simulink model "RBDmodel"  (R2023a)
settings: Solver=ode15s  StartTime=0.0  StopTime=4  FixedStep=0.0001  RelTol=1e-3  AbsTol=1e-3  EnableMultiTasking=on
model workspace (MAT data in the model file):
  C_Gimbal = 0.5
  C_IAP = 0.01
  IAP_Pa = 0
  K_Gimbal = 0
  K_IAP = 200
  LeftAbdominalMuscleForce = 0
  LeftBackMuscleForce = 0
  LeftTransverse1MuscleForce = 0
  LeftTransverse2MuscleForce = 0
  Moment_AR = 0
  Moment_FE = 7.5
  Moment_LB = 0
  RightAbdominalMuscleForce = 0
  RightBackMuscleForce = 0
  RightTransverse1MuscleForce = 0
  RightTransverse2MuscleForce = 0
  a = 1
  b = 1
  muscle_color = [0 0 1]
  muscle_radius = 1
undefined symbols (not defined in the file): X, Y, Z
libraries: nesl_utility x346, sm_lib x329, simulink_extras x33, checkpacklib x3, simulink x1
(part 8 of 12)

== system RBDmodel/main_model/L5 ==
  AR torque feedback L5 : Subsystem
  FE torque feedback L5 : Subsystem
  File Solid : sm_lib/Body Elements/File Solid  ExtGeomFileName=C:\Users\siril\OneDrive\Desktop\TIM-Control\Matlab\Simscape models\CAD - with COM\SymmetricModel\draft7\L5.step  UnitType=FromFile  ExtGeomFileUnits=m  StepReaderType=HEX  ExportConvexHullGeometry=off  InertiaType=CalculateFromGeometry  Mass=1  MassUnits=kg  CenterOfMass=[0 0 0]  CenterOfMassUnits=m  MomentsOfInertia=[1 1 1]  MomentsOfInertiaUnits=kg*m^2  ProductsOfInertia=[0 0 0]  ProductsOfInertiaUnits=kg*m^2  BasedOnType=Density  Density=0.182  DensityUnits=g/cm^3  DoExposeReferenceFrame=on  SerializedFrames=<Frames><Frame><Id>Frame1</Id><Value><Name>To Sacrum</Name><Origin><Source>GeometricFeature</Source><FeatureName>planar surface 1973</FeatureName></Origin><PrimaryAxis><DefinedDirection>+Z</DefinedDirection><Source>GeometricFeature</Source><SourceDirection>+Z</SourceDirection><FeatureName>planar surface 1973</FeatureName></PrimaryAxis><SecondaryAxis><DefinedDirection>+X</DefinedDirection><Source>ReferenceFrame</Source><SourceDirection>+X</SourceDirection><FeatureName></FeatureName></SecondaryAxis></Value></Frame><Frame><Id>Frame2</Id><Value><Name>To L4</Name><Origin><Source>GeometricFeature</Source><FeatureName>planar surface 1977</FeatureName></Origin><PrimaryAxis><DefinedDirection>+Z</DefinedDirection><Source>GeometricFeature</Source><SourceDirection>+Z</SourceDirection><FeatureName>planar surface 1977</FeatureName></PrimaryAxis><SecondaryAxis><DefinedDirection>+X</DefinedDirection><Source>ReferenceFrame</Source><SourceDirection>+X</SourceDirection><FeatureName></FeatureName></SecondaryAxis></Value></Frame><Frame><Id>Frame3</Id><Value><Name>L5 COM</Name><Origin><Source>CenterOfMassFrame</Source><FeatureName></FeatureName></Origin><PrimaryAxis><DefinedDirection>+Z</DefinedDirection><Source>ReferenceFrame</Source><SourceDirection>+Z</SourceDirection><FeatureName></FeatureName></PrimaryAxis><SecondaryAxis><DefinedDirection>+X</DefinedDirection><Source>ReferenceFrame</Source><SourceDirection>+X</SourceDirection><FeatureName></FeatureName></SecondaryAxis></Value></Frame><Frame><Id>Frame4</Id><Value><Name>L5 Abd Force</Name><Origin><Source>GeometricFeature</Source><FeatureName>point 2</FeatureName></Origin><PrimaryAxis><DefinedDirection>+Z</DefinedDirection><Source>GeometricFeature</Source><SourceDirection>+Z</SourceDirection><FeatureName>conical surface 1</FeatureName></PrimaryAxis><SecondaryAxis><DefinedDirection>+X</DefinedDirection><Source>ReferenceFrame</Source><SourceDirection>+X</SourceDirection><FeatureName></FeatureName></SecondaryAxis></Value></Frame><Frame><Id>Frame5</Id><Value><Name>To L4 ISL</Name><Origin><Source>GeometricFeature</Source><FeatureName>point 104</FeatureName></Origin><PrimaryAxis><DefinedDirection>+Z</DefinedDirection><Source>ReferenceFrame</Source><SourceDirection>+Z</SourceDirection><FeatureName></FeatureName></PrimaryAxis><SecondaryAxis><DefinedDirection>+X</DefinedDirection><Source>ReferenceFrame</Source><SourceDirection>+X</SourceDirection><FeatureName></FeatureName></SecondaryAxis></Value></Frame><Frame><Id>Frame6</Id><Value><Name>To S1 ISL</Name><Origin><Source>GeometricFeature</Source><FeatureName>point 11405</FeatureName></Origin><PrimaryAxis><DefinedDirection>+Z</DefinedDirection><Source>ReferenceFrame</Source><SourceDirection>+Z</SourceDirection><FeatureName></FeatureName></PrimaryAxis><SecondaryAxis><DefinedDirection>+X</DefinedDirection><Source>ReferenceFrame</Source><SourceDirection>+X</SourceDirection><FeatureName></FeatureName></SecondaryAxis></Value></Frame><Frame><Id>Frame7</Id><Value><Name>To S1 SSL</Name><Origin><Source>GeometricFeature</Source><FeatureName>point 8728</FeatureName></Origin><PrimaryAxis><DefinedDirection>+Z</DefinedDirection><Source>ReferenceFrame</Source><SourceDirection>+Z</SourceDirection><FeatureName></FeatureName></PrimaryAxis><SecondaryAxis><DefinedDirection>+X</DefinedDirection><Source>ReferenceFrame</Source><SourceDirection>+X</SourceDirection><FeatureName></FeatureName></SecondaryAxis></Value></Frame><Frame><Id>Frame8</Id><Value><Name>To L4 SSL</Name><Origin><Source>GeometricFeature</Source><FeatureName>point 5958</FeatureName></Origin><PrimaryAxis><DefinedDirection>+Z</DefinedDirection><Source>ReferenceFrame</Source><SourceDirection>+Z</SourceDirection><FeatureName></FeatureName></PrimaryAxis><SecondaryAxis><DefinedDirection>+X</DefinedDirection><Source>ReferenceFrame</Source><SourceDirection>+X</SourceDirection><FeatureName></FeatureName></SecondaryAxis></Value></Frame><Frame><Id>Frame9</Id><Value><Name>To Left S1 ITL</Name><Origin><Source>GeometricFeature</Source><FeatureName>point 9071</FeatureName></Origin><PrimaryAxis><DefinedDirection>+Z</DefinedDirection><Source>ReferenceFrame</Source><SourceDirection>+Z</SourceDirection><FeatureName></FeatureName></PrimaryAxis><SecondaryAxis><DefinedDirection>+X</DefinedDirection><Source>ReferenceFrame</Source><SourceDirection>+X</SourceDirection><FeatureName></FeatureName></SecondaryAxis></Value></Frame><Frame><Id>Frame10</Id><Value><Name>To Right S1 ITL</Name><Origin><Source>GeometricFeature</Source><FeatureName>point 3312</FeatureName></Origin><PrimaryAxis><DefinedDirection>+Z</DefinedDirection><Source>ReferenceFrame</Source><SourceDirection>+Z</SourceDirection><FeatureName></FeatureName></PrimaryAxis><SecondaryAxis><DefinedDirection>+X</DefinedDirection><Source>ReferenceFrame</Source><SourceDirection>+X</SourceDirection><FeatureName></FeatureName></SecondaryAxis></Value></Frame><Frame><Id>Frame11</Id><Value><Name>To Left L4 ITL</Name><Origin><Source>GeometricFeature</Source><FeatureName>point 10699</FeatureName></Origin><PrimaryAxis><DefinedDirection>+Z</DefinedDirection><Source>ReferenceFrame</Source><SourceDirection>+Z</SourceDirection><FeatureName></FeatureName></PrimaryAxis><SecondaryAxis><DefinedDirection>+X</DefinedDirection><Source>ReferenceFrame</Source><SourceDirection>+X</SourceDirection><FeatureName></FeatureName></SecondaryAxis></Value></Frame><Frame><Id>Frame12</Id><Value><Name>To Right L4 ITL</Name><Origin><Source>GeometricFeature</Source><FeatureName>point 5014</FeatureName></Origin><PrimaryAxis><DefinedDirection>+Z</DefinedDirection><Source>ReferenceFrame</Source><SourceDirection>+Z</SourceDirection><FeatureName></FeatureName></PrimaryAxis><SecondaryAxis><DefinedDirection>+X</DefinedDirection><Source>ReferenceFrame</Source><SourceDirection>+X</SourceDirection><FeatureName></FeatureName></SecondaryAxis></Value></Frame></Frames>  GraphicType=FromGeometry  MarkerShape=Sphere  MarkerSize=10  GraphicVisPropType=SimpleVisualProperties  GraphicDiffuseColor=[0.8901961 0.85490197 0.7882353]  GraphicSpecularColor=[0.5 0.5 0.5 1.0]  GraphicAmbientColor=[0.15 0.15 0.15 1.0]  GraphicEmissiveColor=[0.0 0.0 0.0 1.0]  GraphicShininess=75  GraphicOpacity=1.0
  Gimbal Joint : sm_lib/Joints/Gimbal Joint  JointMode=Normal  SenseConstraintForce=on  SenseConstraintForceX=off  SenseConstraintForceY=off  SenseConstraintForceZ=off  SenseConstraintTorque=off  SenseConstraintTorqueX=off  SenseConstraintTorqueY=off  SenseConstraintTorqueZ=off  SenseTotalForce=on  SenseTotalForceX=off  SenseTotalForceY=off  SenseTotalForceZ=off  SenseTotalTorque=off  SenseTotalTorqueX=off  SenseTotalTorqueY=off  SenseTotalTorqueZ=off  CompositeWrenchDir=FollowerOnBase  CompositeWrenchFrame=BaseFrame  RxEquilibriumPosition=0  RxEquilibriumPositionUnits=deg  RxSpringStiffness=K_Gimbal  RxSpringStiffnessUnits=N*m/deg  RxDampingCoefficient=C_Gimbal  RxDampingCoefficientUnits=N*m/(deg/s)  RxTorqueActuationMode=InputTorque  RxMotionActuationMode=ComputedMotion  RxSensePosition=on  RxSenseVelocity=off  RxSenseAcceleration=off  RxSenseTorqueForce=on  RxSenseLowerLimitTorqueForce=off  RxSenseUpperLimitTorqueForce=off  RxLowerLimitSpecify=on  RxLowerLimitBound=-30  RxLowerLimitBoundUnits=deg  RxLowerLimitStiffness=10000  RxLowerLimitStiffnessUnits=N*m/deg  RxLowerLimitDamping=100  RxLowerLimitDampingUnits=N*m/(deg/s)  RxLowerLimitTransitionRegionWidth=0.1  RxLowerLimitTransitionRegionWidthUnits=deg  RxUpperLimitSpecify=on  RxUpperLimitBound=30  RxUpperLimitBoundUnits=deg  RxUpperLimitStiffness=10000  RxUpperLimitStiffnessUnits=N*m/deg  RxUpperLimitDamping=100  RxUpperLimitDampingUnits=N*m/(deg/s)  RxUpperLimitTransitionRegionWidth=0.1  RxUpperLimitTransitionRegionWidthUnits=deg  RxPositionTargetSpecify=off  RxPositionTargetPriority=High  RxPositionTargetValue=0  RxPositionTargetValueUnits=deg  RxVelocityTargetSpecify=off  RxVelocityTargetPriority=High  RxVelocityTargetValue=0  RxVelocityTargetValueUnits=deg/s  RyEquilibriumPosition=0  RyEquilibriumPositionUnits=deg  RySpringStiffness=K_Gimbal  RySpringStiffnessUnits=N*m/deg  RyDampingCoefficient=C_Gimbal  RyDampingCoefficientUnits=N*m/(deg/s)  RyTorqueActuationMode=InputTorque  RyMotionActuationMode=ComputedMotion  RySensePosition=on  RySenseVelocity=off  RySenseAcceleration=off  RySenseTorqueForce=on  RySenseLowerLimitTorqueForce=off  RySenseUpperLimitTorqueForce=off  RyLowerLimitSpecify=on  RyLowerLimitBound=-30  RyLowerLimitBoundUnits=deg  RyLowerLimitStiffness=10000  RyLowerLimitStiffnessUnits=N*m/deg  RyLowerLimitDamping=100  RyLowerLimitDampingUnits=N*m/(deg/s)  RyLowerLimitTransitionRegionWidth=0.1  RyLowerLimitTransitionRegionWidthUnits=deg  RyUpperLimitSpecify=on  RyUpperLimitBound=30  RyUpperLimitBoundUnits=deg  RyUpperLimitStiffness=10000  RyUpperLimitStiffnessUnits=N*m/deg  RyUpperLimitDamping=100  RyUpperLimitDampingUnits=N*m/(deg/s)  RyUpperLimitTransitionRegionWidth=0.1  RyUpperLimitTransitionRegionWidthUnits=deg  RyPositionTargetSpecify=off  RyPositionTargetPriority=High  RyPositionTargetValue=0  RyPositionTargetValueUnits=deg  RyVelocityTargetSpecify=off  RyVelocityTargetPriority=High  RyVelocityTargetValue=0  RyVelocityTargetValueUnits=deg/s  RzEquilibriumPosition=0  RzEquilibriumPositionUnits=deg  RzSpringStiffness=K_Gimbal  RzSpringStiffnessUnits=N*m/deg  RzDampingCoefficient=C_Gimbal  RzDampingCoefficientUnits=N*m/(deg/s)  RzTorqueActuationMode=InputTorque  RzMotionActuationMode=ComputedMotion  RzSensePosition=on  RzSenseVelocity=off  RzSenseAcceleration=off  RzSenseTorqueForce=on  RzSenseLowerLimitTorqueForce=off  RzSenseUpperLimitTorqueForce=off  RzLowerLimitSpecify=on  RzLowerLimitBound=-30  RzLowerLimitBoundUnits=deg  RzLowerLimitStiffness=10000  RzLowerLimitStiffnessUnits=N*m/deg  RzLowerLimitDamping=100  RzLowerLimitDampingUnits=N*m/(deg/s)  RzLowerLimitTransitionRegionWidth=0.1  RzLowerLimitTransitionRegionWidthUnits=deg  RzUpperLimitSpecify=on  RzUpperLimitBound=30  RzUpperLimitBoundUnits=deg  RzUpperLimitStiffness=10000  RzUpperLimitStiffnessUnits=N*m/deg  RzUpperLimitDamping=100  RzUpperLimitDampingUnits=N*m/(deg/s)  RzUpperLimitTransitionRegionWidth=0.1  RzUpperLimitTransitionRegionWidthUnits=deg  RzPositionTargetSpecify=off  RzPositionTargetPriority=High  RzPositionTargetValue=0  RzPositionTargetValueUnits=deg  RzVelocityTargetSpecify=off  RzVelocityTargetPriority=High  RzVelocityTargetValue=0  RzVelocityTargetValueUnits=deg/s
  LB torque feedback L5 : Subsystem
  to sacrum : PMIOPort  Side=Left
  to L4 : PMIOPort  Port=2  Side=Right
  FE torque : PMIOPort  Port=3  Side=Right
  FE rot : PMIOPort  Port=4  Side=Right
  LB rot : PMIOPort  Port=5  Side=Right
  LB torque : PMIOPort  Port=6  Side=Right
  AR rot : PMIOPort  Port=7  Side=Right
  AR torque : PMIOPort  Port=8  Side=Right
  L5 COM : PMIOPort  Port=9  Side=Right
  L5 Abd Force : PMIOPort  Port=10  Side=Right
  To L4 ISL : PMIOPort  Port=11  Side=Right
  To S1 ISL : PMIOPort  Port=12  Side=Right
  To L4 SSL : PMIOPort  Port=13  Side=Right
  To S1 SSL : PMIOPort  Port=14  Side=Right
  To Left S1 ITL : PMIOPort  Port=15  Side=Right
  To Right S1 ITL : PMIOPort  Port=16  Side=Right
  To Left L4 ITL : PMIOPort  Port=17  Side=Right
  To Right L4 ITL : PMIOPort  Port=18  Side=Right
  connections:
  File Solid/LConn2 -- to L4/RConn1
  to sacrum/RConn1 -- Gimbal Joint/LConn1
  Gimbal Joint/RConn1 -- File Solid/LConn1
  Gimbal Joint/LConn2 -- FE torque feedback L5/RConn1
  Gimbal Joint/LConn3 -- LB torque feedback L5/RConn1
  Gimbal Joint/LConn4 -- AR torque feedback L5/RConn1
  Gimbal Joint/RConn2 -- FE torque feedback L5/LConn1 -- FE rot/RConn1
  Gimbal Joint/RConn4 -- LB torque feedback L5/LConn1 -- LB rot/RConn1
  Gimbal Joint/RConn6 -- AR rot/RConn1 -- AR torque feedback L5/LConn1
  FE torque/RConn1 -- Gimbal Joint/RConn3
  LB torque/RConn1 -- Gimbal Joint/RConn5
  AR torque/RConn1 -- Gimbal Joint/RConn7
  L5 COM/RConn1 -- File Solid/RConn2
  L5 Abd Force/RConn1 -- File Solid/LConn3
  To L4 ISL/RConn1 -- File Solid/RConn3
  To S1 ISL/RConn1 -- File Solid/LConn4
  To S1 SSL/RConn1 -- File Solid/RConn4
  To L4 SSL/RConn1 -- File Solid/LConn5
  To Left S1 ITL/RConn1 -- File Solid/RConn5
  To Right S1 ITL/RConn1 -- File Solid/LConn6
  To Left L4 ITL/RConn1 -- File Solid/RConn6
  To Right L4 ITL/RConn1 -- File Solid/LConn7

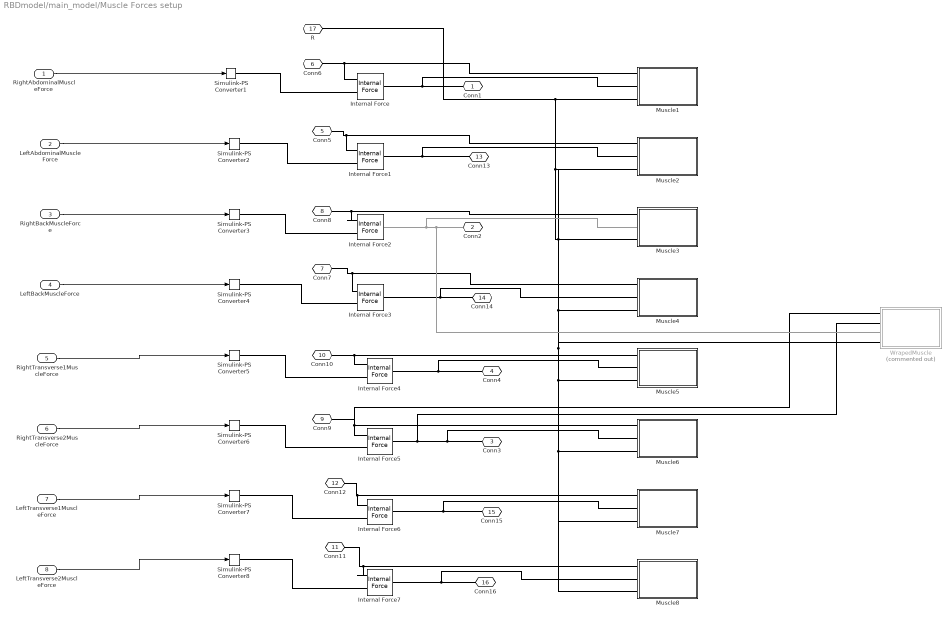
== system RBDmodel/main_model/Muscle Forces setup ==
  RightAbdominalMuscleForce : Inport
  LeftAbdominalMuscleForce : Inport  Port=2
  RightBackMuscleForce : Inport  Port=3
  LeftBackMuscleForce : Inport  Port=4
  RightTransverse1MuscleForce : Inport  Port=5
  RightTransverse2MuscleForce : Inport  Port=6
  LeftTransverse1MuscleForce : Inport  Port=7
  LeftTransverse2MuscleForce : Inport  Port=8
  Internal Force{,1..7} (8 alike) : sm_lib/Forces and Torques/Internal Force
  Muscle1 : Subsystem
  Muscle2 : Subsystem
  Muscle3 : Subsystem
  Muscle4 : Subsystem
  Muscle5 : Subsystem
  Muscle6 : Subsystem
  Muscle7 : Subsystem
  Muscle8 : Subsystem
  Simulink-PS Converter{1..8} (8 alike) : nesl_utility/Simulink-PS Converter  PhysicalDomain=network_engine_domain  SubClassName=ps_input  LeftPortType=input  RightPortType=output  PseudoPeriodic=off  Frequencies=[]  NoiseDistribution=none  NoiseParameters=[]  Unit=1  AffineConversion=off  FilteringAndDerivatives=provide  SimscapeFilterOrder=1  InputFilterTimeConstant=0.001  UdotUserProvided=0
  WrapedMuscle : Subsystem  Commented=on
  Conn1 : PMIOPort  Side=Right
  Conn2 : PMIOPort  Port=2  Side=Right
  Conn3 : PMIOPort  Port=3  Side=Right
  Conn4 : PMIOPort  Port=4  Side=Right
  Conn5 : PMIOPort  Port=5  Side=Left
  Conn6 : PMIOPort  Port=6  Side=Left
  Conn7 : PMIOPort  Port=7  Side=Left
  Conn8 : PMIOPort  Port=8  Side=Left
  Conn9 : PMIOPort  Port=9  Side=Left
  Conn10 : PMIOPort  Port=10  Side=Left
  Conn11 : PMIOPort  Port=11  Side=Left
  Conn12 : PMIOPort  Port=12  Side=Left
  Conn13 : PMIOPort  Port=13  Side=Right
  Conn14 : PMIOPort  Port=14  Side=Right
  Conn15 : PMIOPort  Port=15  Side=Right
  Conn16 : PMIOPort  Port=16  Side=Right
  R : PMIOPort  Port=17  Side=Left
  wires:
  LeftTransverse2MuscleForce/1 -> Simulink-PS Converter8/1
  RightBackMuscleForce/1 -> Simulink-PS Converter3/1
  RightTransverse1MuscleForce/1 -> Simulink-PS Converter5/1
  LeftTransverse1MuscleForce/1 -> Simulink-PS Converter7/1
  RightTransverse2MuscleForce/1 -> Simulink-PS Converter6/1
  LeftAbdominalMuscleForce/1 -> Simulink-PS Converter2/1
  RightAbdominalMuscleForce/1 -> Simulink-PS Converter1/1
  LeftBackMuscleForce/1 -> Simulink-PS Converter4/1
  connections:
  Muscle4/RConn1 -- Conn7/RConn1 -- Internal Force3/LConn1
  Conn9/RConn1 -- WrapedMuscle/RConn1 -- Muscle6/RConn1 -- Internal Force5/LConn1
  Muscle8/RConn3 -- Muscle7/RConn3 -- Muscle6/RConn3 -- Muscle5/RConn3 -- WrapedMuscle/RConn4 -- Muscle4/RConn3 -- Muscle3/RConn3 -- Muscle2/RConn3 -- R/RConn1 -- Muscle1/RConn3
  Muscle4/RConn2 -- Conn14/RConn1 -- Internal Force3/RConn1
  Muscle5/RConn1 -- Conn10/RConn1 -- Internal Force4/LConn1
  Muscle6/RConn2 -- Conn3/RConn1 -- WrapedMuscle/RConn2 -- Internal Force5/RConn1
  Muscle7/RConn1 -- Conn12/RConn1 -- Internal Force6/LConn1
  Internal Force7/LConn1 -- Conn11/RConn1 -- Muscle8/RConn1
  Simulink-PS Converter8/RConn1 -- Internal Force7/LConn2
  Muscle2/RConn1 -- Conn5/RConn1 -- Internal Force1/LConn1
  Simulink-PS Converter2/RConn1 -- Internal Force1/LConn2
  Muscle7/RConn2 -- Conn15/RConn1 -- Internal Force6/RConn1
  Muscle2/RConn2 -- Conn13/RConn1 -- Internal Force1/RConn1
  Simulink-PS Converter1/RConn1 -- Internal Force/LConn2
  WrapedMuscle/RConn3 -- Conn2/RConn1 -- Muscle3/RConn2 -- Internal Force2/RConn1
  Muscle1/RConn1 -- Conn6/RConn1 -- Internal Force/LConn1
  Simulink-PS Converter3/RConn1 -- Internal Force2/LConn2
  Simulink-PS Converter7/RConn1 -- Internal Force6/LConn2
  Internal Force2/LConn1 -- Conn8/RConn1 -- Muscle3/RConn1
  Muscle1/RConn2 -- Conn1/RConn1 -- Internal Force/RConn1
  Simulink-PS Converter5/RConn1 -- Internal Force4/LConn2
  Muscle8/RConn2 -- Conn16/RConn1 -- Internal Force7/RConn1
  Muscle5/RConn2 -- Conn4/RConn1 -- Internal Force4/RConn1
  Simulink-PS Converter4/RConn1 -- Internal Force3/LConn2
  Simulink-PS Converter6/RConn1 -- Internal Force5/LConn2

== system RBDmodel/main_model/Plumbline setup ==
  Gain : Gain  Gain=100
  Gain1 : Gain  Gain=100
  Gain2 : Gain  Gain=100
  PS-Simulink Converter2 : nesl_utility/PS-Simulink Converter  PhysicalDomain=network_engine_domain  SubClassName=ps_output  LeftPortType=input  RightPortType=output  PseudoPeriodic=off  Frequencies=[]  VectorFormat=inherit  Unit=inherit  AffineConversion=off
  PS-Simulink Converter3 : nesl_utility/PS-Simulink Converter  PhysicalDomain=network_engine_domain  SubClassName=ps_output  LeftPortType=input  RightPortType=output  PseudoPeriodic=off  Frequencies=[]  VectorFormat=inherit  Unit=inherit  AffineConversion=off
  PS-Simulink Converter4 : nesl_utility/PS-Simulink Converter  PhysicalDomain=network_engine_domain  SubClassName=ps_output  LeftPortType=input  RightPortType=output  PseudoPeriodic=off  Frequencies=[]  VectorFormat=inherit  Unit=inherit  AffineConversion=off
  T1-S1 Bushing Joint : sm_lib/Joints/Bushing Joint  JointMode=Normal  SenseConstraintForce=off  SenseConstraintForceX=off  SenseConstraintForceY=off  SenseConstraintForceZ=off  SenseConstraintTorque=off  SenseConstraintTorqueX=off  SenseConstraintTorqueY=off  SenseConstraintTorqueZ=off  SenseTotalForce=off  SenseTotalForceX=off  SenseTotalForceY=off  SenseTotalForceZ=off  SenseTotalTorque=off  SenseTotalTorqueX=off  SenseTotalTorqueY=off  SenseTotalTorqueZ=off  CompositeWrenchDir=FollowerOnBase  CompositeWrenchFrame=BaseFrame  PxEquilibriumPosition=0  PxEquilibriumPositionUnits=m  PxSpringStiffness=0  PxSpringStiffnessUnits=N/m  PxDampingCoefficient=0  PxDampingCoefficientUnits=N/(m/s)  PxTorqueActuationMode=NoTorque  PxMotionActuationMode=ComputedMotion  PxSensePosition=on  PxSenseVelocity=off  PxSenseAcceleration=off  PxSenseTorqueForce=off  PxSenseLowerLimitTorqueForce=off  PxSenseUpperLimitTorqueForce=off  PxLowerLimitSpecify=off  PxLowerLimitBound=-1  PxLowerLimitBoundUnits=m  PxLowerLimitStiffness=1e6  PxLowerLimitStiffnessUnits=N/m  PxLowerLimitDamping=1e3  PxLowerLimitDampingUnits=N/(m/s)  PxLowerLimitTransitionRegionWidth=1e-4  PxLowerLimitTransitionRegionWidthUnits=m  PxUpperLimitSpecify=off  PxUpperLimitBound=1  PxUpperLimitBoundUnits=m  PxUpperLimitStiffness=1e6  PxUpperLimitStiffnessUnits=N/m  PxUpperLimitDamping=1e3  PxUpperLimitDampingUnits=N/(m/s)  PxUpperLimitTransitionRegionWidth=1e-4  PxUpperLimitTransitionRegionWidthUnits=m  PxPositionTargetSpecify=off  PxPositionTargetPriority=High  PxPositionTargetValue=0  PxPositionTargetValueUnits=m  PxVelocityTargetSpecify=off  PxVelocityTargetPriority=High  PxVelocityTargetValue=0  PxVelocityTargetValueUnits=m/s  PyEquilibriumPosition=0  PyEquilibriumPositionUnits=m  PySpringStiffness=0  PySpringStiffnessUnits=N/m  PyDampingCoefficient=0  PyDampingCoefficientUnits=N/(m/s)  PyTorqueActuationMode=NoTorque  PyMotionActuationMode=ComputedMotion  PySensePosition=on  PySenseVelocity=off  PySenseAcceleration=off  PySenseTorqueForce=off  PySenseLowerLimitTorqueForce=off  PySenseUpperLimitTorqueForce=off  PyLowerLimitSpecify=off  PyLowerLimitBound=-1  PyLowerLimitBoundUnits=m  PyLowerLimitStiffness=1e6  PyLowerLimitStiffnessUnits=N/m  PyLowerLimitDamping=1e3  PyLowerLimitDampingUnits=N/(m/s)  PyLowerLimitTransitionRegionWidth=1e-4  PyLowerLimitTransitionRegionWidthUnits=m  PyUpperLimitSpecify=off  PyUpperLimitBound=1  PyUpperLimitBoundUnits=m  PyUpperLimitStiffness=1e6  PyUpperLimitStiffnessUnits=N/m  PyUpperLimitDamping=1e3  PyUpperLimitDampingUnits=N/(m/s)  PyUpperLimitTransitionRegionWidth=1e-4  PyUpperLimitTransitionRegionWidthUnits=m  PyPositionTargetSpecify=off  PyPositionTargetPriority=High  PyPositionTargetValue=0  PyPositionTargetValueUnits=m  PyVelocityTargetSpecify=off  PyVelocityTargetPriority=High  PyVelocityTargetValue=0  PyVelocityTargetValueUnits=m/s  PzEquilibriumPosition=0  PzEquilibriumPositionUnits=m  PzSpringStiffness=0  PzSpringStiffnessUnits=N/m  PzDampingCoefficient=0  PzDampingCoefficientUnits=N/(m/s)  PzTorqueActuationMode=NoTorque  PzMotionActuationMode=ComputedMotion  PzSensePosition=on  PzSenseVelocity=off  PzSenseAcceleration=off  PzSenseTorqueForce=off  PzSenseLowerLimitTorqueForce=off  PzSenseUpperLimitTorqueForce=off  PzLowerLimitSpecify=off  PzLowerLimitBound=-1  PzLowerLimitBoundUnits=m  PzLowerLimitStiffness=1e6  PzLowerLimitStiffnessUnits=N/m  PzLowerLimitDamping=1e3  PzLowerLimitDampingUnits=N/(m/s)  PzLowerLimitTransitionRegionWidth=1e-4  PzLowerLimitTransitionRegionWidthUnits=m  PzUpperLimitSpecify=off  PzUpperLimitBound=1  PzUpperLimitBoundUnits=m  PzUpperLimitStiffness=1e6  PzUpperLimitStiffnessUnits=N/m  PzUpperLimitDamping=1e3  PzUpperLimitDampingUnits=N/(m/s)  PzUpperLimitTransitionRegionWidth=1e-4  PzUpperLimitTransitionRegionWidthUnits=m  PzPositionTargetSpecify=off  PzPositionTargetPriority=High  PzPositionTargetValue=0  PzPositionTargetValueUnits=m  PzVelocityTargetSpecify=off  PzVelocityTargetPriority=High  PzVelocityTargetValue=0  PzVelocityTargetValueUnits=m/s  RxEquilibriumPosition=0  RxEquilibriumPositionUnits=deg  RxSpringStiffness=0  RxSpringStiffnessUnits=N*m/deg  RxDampingCoefficient=0  RxDampingCoefficientUnits=N*m/(deg/s)  RxTorqueActuationMode=NoTorque  RxMotionActuationMode=ComputedMotion  RxSensePosition=off  RxSenseVelocity=off  RxSenseAcceleration=off  RxSenseTorqueForce=off  RxSenseLowerLimitTorqueForce=off  RxSenseUpperLimitTorqueForce=off  RxLowerLimitSpecify=off  RxLowerLimitBound=-90  RxLowerLimitBoundUnits=deg  RxLowerLimitStiffness=1e4  RxLowerLimitStiffnessUnits=N*m/deg  RxLowerLimitDamping=10  RxLowerLimitDampingUnits=N*m/(deg/s)  RxLowerLimitTransitionRegionWidth=0.1  RxLowerLimitTransitionRegionWidthUnits=deg  RxUpperLimitSpecify=off  RxUpperLimitBound=90  RxUpperLimitBoundUnits=deg  RxUpperLimitStiffness=1e4  RxUpperLimitStiffnessUnits=N*m/deg  RxUpperLimitDamping=10  RxUpperLimitDampingUnits=N*m/(deg/s)  RxUpperLimitTransitionRegionWidth=0.1  RxUpperLimitTransitionRegionWidthUnits=deg  RxPositionTargetSpecify=off  RxPositionTargetPriority=High  RxPositionTargetValue=0  RxPositionTargetValueUnits=deg  RxVelocityTargetSpecify=off  RxVelocityTargetPriority=High  RxVelocityTargetValue=0  RxVelocityTargetValueUnits=deg/s  RyEquilibriumPosition=0  RyEquilibriumPositionUnits=deg  RySpringStiffness=0  RySpringStiffnessUnits=N*m/deg  RyDampingCoefficient=0  RyDampingCoefficientUnits=N*m/(deg/s)  RyTorqueActuationMode=NoTorque  RyMotionActuationMode=ComputedMotion  RySensePosition=off  RySenseVelocity=off  RySenseAcceleration=off  RySenseTorqueForce=off  RySenseLowerLimitTorqueForce=off  RySenseUpperLimitTorqueForce=off  RyLowerLimitSpecify=off  RyLowerLimitBound=-90  RyLowerLimitBoundUnits=deg  RyLowerLimitStiffness=1e4  RyLowerLimitStiffnessUnits=N*m/deg  RyLowerLimitDamping=10  RyLowerLimitDampingUnits=N*m/(deg/s)  RyLowerLimitTransitionRegionWidth=0.1  RyLowerLimitTransitionRegionWidthUnits=deg  RyUpperLimitSpecify=off  RyUpperLimitBound=90  RyUpperLimitBoundUnits=deg  RyUpperLimitStiffness=1e4  RyUpperLimitStiffnessUnits=N*m/deg  RyUpperLimitDamping=10  RyUpperLimitDampingUnits=N*m/(deg/s)  RyUpperLimitTransitionRegionWidth=0.1  RyUpperLimitTransitionRegionWidthUnits=deg  RyPositionTargetSpecify=off  RyPositionTargetPriority=High  RyPositionTargetValue=0  RyPositionTargetValueUnits=deg  RyVelocityTargetSpecify=off  RyVelocityTargetPriority=High  RyVelocityTargetValue=0  RyVelocityTargetValueUnits=deg/s  RzEquilibriumPosition=0  RzEquilibriumPositionUnits=deg  RzSpringStiffness=0  RzSpringStiffnessUnits=N*m/deg  RzDampingCoefficient=0  RzDampingCoefficientUnits=N*m/(deg/s)  RzTorqueActuationMode=NoTorque  RzMotionActuationMode=ComputedMotion  RzSensePosition=off  RzSenseVelocity=off  RzSenseAcceleration=off  RzSenseTorqueForce=off  RzSenseLowerLimitTorqueForce=off  RzSenseUpperLimitTorqueForce=off  RzLowerLimitSpecify=off  RzLowerLimitBound=-90  RzLowerLimitBoundUnits=deg  RzLowerLimitStiffness=1e4  RzLowerLimitStiffnessUnits=N*m/deg  RzLowerLimitDamping=10  RzLowerLimitDampingUnits=N*m/(deg/s)  RzLowerLimitTransitionRegionWidth=0.1  RzLowerLimitTransitionRegionWidthUnits=deg  RzUpperLimitSpecify=off  RzUpperLimitBound=90  RzUpperLimitBoundUnits=deg  RzUpperLimitStiffness=1e4  RzUpperLimitStiffnessUnits=N*m/deg  RzUpperLimitDamping=10  RzUpperLimitDampingUnits=N*m/(deg/s)  RzUpperLimitTransitionRegionWidth=0.1  RzUpperLimitTransitionRegionWidthUnits=deg  RzPositionTargetSpecify=off  RzPositionTargetPriority=High  RzPositionTargetValue=0  RzPositionTargetValueUnits=deg  RzVelocityTargetSpecify=off  RzVelocityTargetPriority=High  RzVelocityTargetValue=0  RzVelocityTargetValueUnits=deg/s
  Conn1 : PMIOPort  Side=Left
  Conn2 : PMIOPort  Port=2  Side=Right
  x : Outport
  y : Outport  Port=2
  z : Outport  Port=3
  wires:
  PS-Simulink Converter3/1 -> Gain1/1  "y"
  Gain1/1 -> y/1  "y"
  PS-Simulink Converter2/1 -> Gain/1  "x"
  PS-Simulink Converter4/1 -> Gain2/1  "z"
  Gain/1 -> x/1  "x"
  Gain2/1 -> z/1  "z"
  connections:
  PS-Simulink Converter3/LConn1 -- T1-S1 Bushing Joint/RConn3
  PS-Simulink Converter4/LConn1 -- T1-S1 Bushing Joint/RConn4
  PS-Simulink Converter2/LConn1 -- T1-S1 Bushing Joint/RConn2
  Conn1/RConn1 -- T1-S1 Bushing Joint/LConn1
  T1-S1 Bushing Joint/RConn1 -- Conn2/RConn1

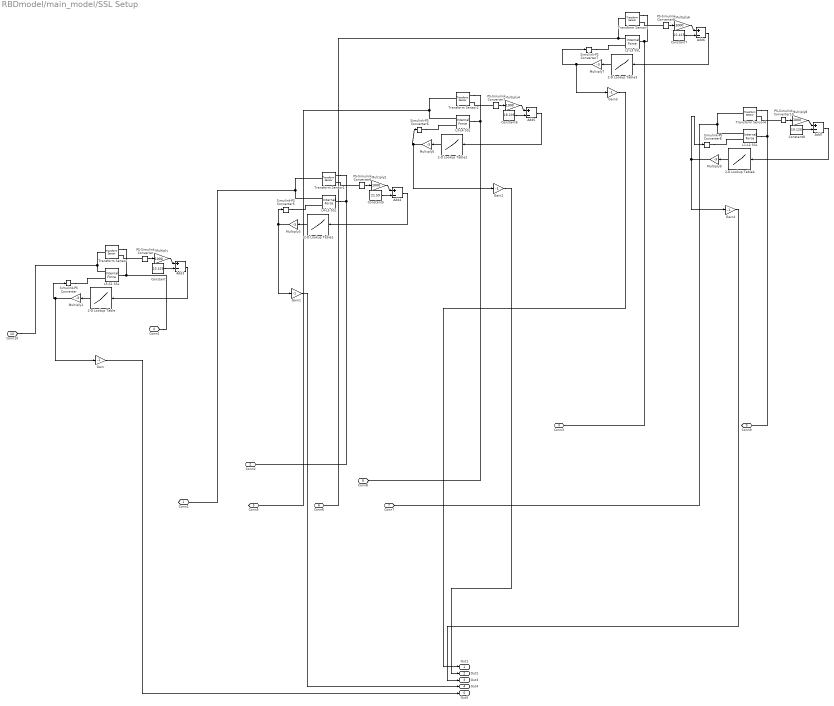
== system RBDmodel/main_model/SSL Setup ==
  2-D Lookup Table : Lookup_n-D  NumberOfTableDimensions=1  BreakpointsForDimension1=[0;0.272;4.08;5.984;7.888]  BreakpointsForDimension2=[1:3]  Table=[0;0;8.4;21;84]  InternalRulePriority=Speed  RndMeth=Simplest
  2-D Lookup Table1 : Lookup_n-D  NumberOfTableDimensions=1  BreakpointsForDimension1=[0;0.223;3.345;4.906;6.467]  BreakpointsForDimension2=[1:3]  Table=[0;0;8.4;21;84]  InternalRulePriority=Speed  RndMeth=Simplest
  2-D Lookup Table2 : Lookup_n-D  NumberOfTableDimensions=1  BreakpointsForDimension1=[0;0.194;2.91;4.268;5.626]  BreakpointsForDimension2=[1:3]  Table=[0;0;8.4;21;84]  InternalRulePriority=Speed  RndMeth=Simplest
  2-D Lookup Table3 : Lookup_n-D  NumberOfTableDimensions=1  BreakpointsForDimension1=[0;0.268;4.02;5.896;7.772]  BreakpointsForDimension2=[1:3]  Table=[0;0;8.4;21;84]  InternalRulePriority=Speed  RndMeth=Simplest
  2-D Lookup Table4 : Lookup_n-D  NumberOfTableDimensions=1  BreakpointsForDimension1=[0;0.223;3.345;4.906;6.467]  BreakpointsForDimension2=[1:3]  Table=[0;0;8.4;21;84]  InternalRulePriority=Speed  RndMeth=Simplest
  Add{3..7} (5 alike) : Sum  Inputs=+-
  Constant : Constant  Value=23.426
  Constant5 : Constant  Value=21.59
  Constant6 : Constant  Value=18.205
  Constant7 : Constant  Value=21.415
  Constant8 : Constant  Value=19.125
  Gain{,1..4} (5 alike) : Gain  Gain=-1
  L1-L2 SSL : sm_lib/Forces and Torques/Internal Force
  L2-L3 SSL : sm_lib/Forces and Torques/Internal Force
  L3-L4 SSL : sm_lib/Forces and Torques/Internal Force
  L4-L5 SSL : sm_lib/Forces and Torques/Internal Force
  L5-S1 SSL : sm_lib/Forces and Torques/Internal Force
  Multiply{,2,4,6,8} (5 alike) : Gain  Gain=1000
  Multiply{1,3,5,7,9} (5 alike) : Gain  Gain=-3
  PS-Simulink Converter{,6..8,10} (5 alike) : nesl_utility/PS-Simulink Converter  PhysicalDomain=network_engine_domain  SubClassName=ps_output  LeftPortType=input  RightPortType=output  PseudoPeriodic=off  Frequencies=[]  VectorFormat=inherit  Unit=inherit  AffineConversion=off
  Simulink-PS Converter{,5..8} (5 alike) : nesl_utility/Simulink-PS Converter  PhysicalDomain=network_engine_domain  SubClassName=ps_input  LeftPortType=input  RightPortType=output  PseudoPeriodic=off  Frequencies=[]  NoiseDistribution=none  NoiseParameters=[]  Unit=1  AffineConversion=off  FilteringAndDerivatives=provide  SimscapeFilterOrder=1  InputFilterTimeConstant=0.001  UdotUserProvided=0
  Transform Sensor{,1..4} (5 alike) : sm_lib/Frames and Transforms/Transform Sensor  MeasurementFrame=World  RotationSequence=XYX  SenseAngle=off  SenseAxis=off  SenseQ=off  SenseR=off  SenseRotationSequence=off  SenseOmegaX=off  SenseOmegaY=off  SenseOmegaZ=off  SenseQDot=off  SenseRDot=off  SenseRotationSequenceDot=off  SenseAlphaX=off  SenseAlphaY=off  SenseAlphaZ=off  SenseQDDot=off  SenseRDDot=off  SenseX=off  SenseY=off  SenseZ=off  SenseRad=off  SenseAzim=off  SenseDist=on  SenseInc=off  SenseXDot=off  SenseYDot=off  SenseZDot=off  SenseRadDot=off  SenseAzimDot=off  SenseDistDot=off  SenseIncDot=off  SenseXDDot=off  SenseYDDot=off  SenseZDDot=off  SenseRadDDot=off  SenseAzimDDot=off  SenseDistDDot=off  SenseIncDDot=off
  Conn1 : PMIOPort  Side=Left
  Conn2 : PMIOPort  Port=2  Side=Left
  Conn3 : PMIOPort  Port=3  Side=Left
  Conn4 : PMIOPort  Port=4  Side=Left
  Conn5 : PMIOPort  Port=5  Side=Left
  Conn6 : PMIOPort  Port=6  Side=Left
  Conn7 : PMIOPort  Port=7  Side=Left
  Conn8 : PMIOPort  Port=8  Side=Left
  Conn9 : PMIOPort  Port=9  Side=Left
  Conn10 : PMIOPort  Port=10  Side=Left
  Out1 : Outport
  Out2 : Outport  Port=2
  Out3 : Outport  Port=3
  Out4 : Outport  Port=4
  Out5 : Outport  Port=5
  wires:
  PS-Simulink Converter10/1 -> Multiply8/1
  Multiply1/1 -> Gain/1, Simulink-PS Converter/1
  PS-Simulink Converter/1 -> Multiply/1
  2-D Lookup Table/1 -> Multiply1/1
  Constant6/1 -> Add5/2
  Add6/1 -> 2-D Lookup Table3/1
  2-D Lookup Table2/1 -> Multiply5/1
  Multiply7/1 -> Gain3/1, Simulink-PS Converter7/1
  Multiply8/1 -> Add7/1
  2-D Lookup Table1/1 -> Multiply3/1
  Gain1/1 -> Out4/1
  Multiply4/1 -> Add5/1
  PS-Simulink Converter8/1 -> Multiply6/1
  Gain2/1 -> Out2/1
  Constant8/1 -> Add7/2
  Add5/1 -> 2-D Lookup Table2/1
  Multiply3/1 -> Simulink-PS Converter5/1, Gain1/1
  Add3/1 -> 2-D Lookup Table/1
  Constant/1 -> Add3/2
  2-D Lookup Table3/1 -> Multiply7/1
  Multiply6/1 -> Add6/1
  Constant5/1 -> Add4/2
  PS-Simulink Converter6/1 -> Multiply2/1
  Multiply5/1 -> Gain2/1, Simulink-PS Converter6/1
  Constant7/1 -> Add6/2
  2-D Lookup Table4/1 -> Multiply9/1
  Add4/1 -> 2-D Lookup Table1/1
  Multiply/1 -> Add3/1
  Multiply9/1 -> Gain4/1, Simulink-PS Converter8/1
  Multiply2/1 -> Add4/1
  PS-Simulink Converter7/1 -> Multiply4/1
  Gain/1 -> Out5/1
  Add7/1 -> 2-D Lookup Table4/1
  Gain3/1 -> Out1/1
  Gain4/1 -> Out3/1
  connections:
  Simulink-PS Converter8/RConn1 -- L1-L2 SSL/LConn2
  L5-S1 SSL/RConn1 -- Conn4/RConn1 -- Transform Sensor/RConn1
  Simulink-PS Converter7/RConn1 -- L2-L3 SSL/LConn2
  L3-L4 SSL/LConn1 -- Conn5/RConn1 -- Transform Sensor2/LConn1
  L4-L5 SSL/LConn1 -- Conn1/RConn1 -- Transform Sensor1/LConn1
  L2-L3 SSL/LConn1 -- Conn6/RConn1 -- Transform Sensor3/LConn1
  PS-Simulink Converter8/LConn1 -- Transform Sensor3/RConn2
  Simulink-PS Converter/RConn1 -- L5-S1 SSL/LConn2
  Simulink-PS Converter6/RConn1 -- L3-L4 SSL/LConn2
  L5-S1 SSL/LConn1 -- Conn10/RConn1 -- Transform Sensor/LConn1
  PS-Simulink Converter7/LConn1 -- Transform Sensor2/RConn2
  PS-Simulink Converter6/LConn1 -- Transform Sensor1/RConn2
  L4-L5 SSL/RConn1 -- Conn2/RConn1 -- Transform Sensor1/RConn1
  L1-L2 SSL/LConn1 -- Conn7/RConn1 -- Transform Sensor4/LConn1
  Transform Sensor2/RConn1 -- Conn8/RConn1 -- L3-L4 SSL/RConn1
  L2-L3 SSL/RConn1 -- Conn3/RConn1 -- Transform Sensor3/RConn1
  L1-L2 SSL/RConn1 -- Conn9/RConn1 -- Transform Sensor4/RConn1
  Simulink-PS Converter5/RConn1 -- L4-L5 SSL/LConn2
  PS-Simulink Converter/LConn1 -- Transform Sensor/RConn2
  PS-Simulink Converter10/LConn1 -- Transform Sensor4/RConn2

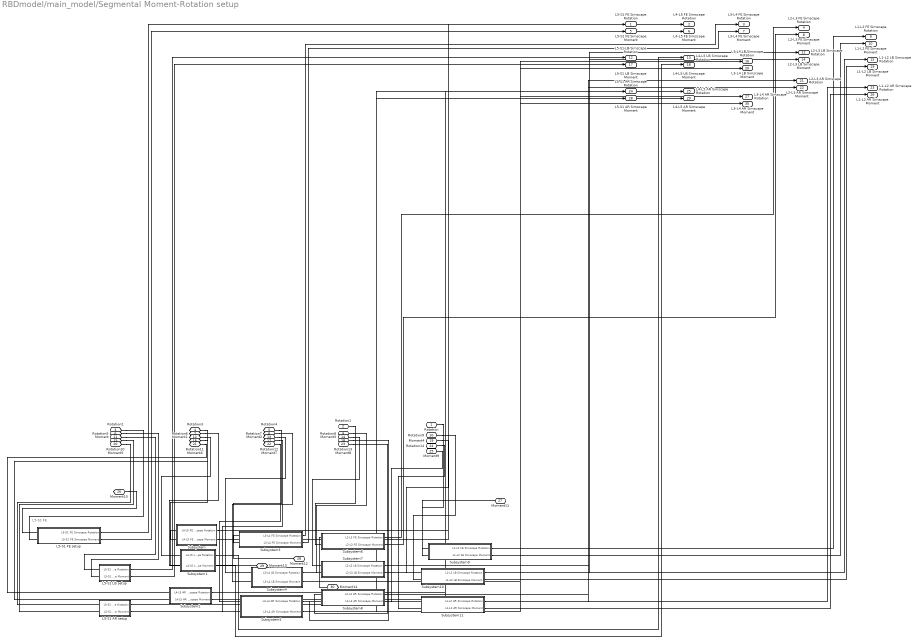
== system RBDmodel/main_model/Segmental Moment-Rotation setup ==
  note: L5-S1 FE
  L5-S1 AR setup : Subsystem
  L5-S1 FE setup : Subsystem
  L5-S1 LB setup : Subsystem
  Subsystem : Subsystem
  Subsystem1 : Subsystem
  Subsystem10 : Subsystem
  Subsystem11 : Subsystem
  Subsystem2 : Subsystem
  Subsystem3 : Subsystem
  Subsystem4 : Subsystem
  Subsystem5 : Subsystem
  Subsystem6 : Subsystem
  Subsystem7 : Subsystem
  Subsystem8 : Subsystem
  Subsystem9 : Subsystem
  Rotation : PMIOPort  Side=Left
  Rotation1 : PMIOPort  Port=2  Side=Left
  Rotation2 : PMIOPort  Port=3  Side=Left
  Rotation3 : PMIOPort  Port=4  Side=Left
  Rotation4 : PMIOPort  Port=5  Side=Left
  Rotation5 : PMIOPort  Port=6  Side=Left
  Rotation6 : PMIOPort  Port=7  Side=Left
  Rotation7 : PMIOPort  Port=8  Side=Left
  Rotation8 : PMIOPort  Port=9  Side=Left
  Rotation9 : PMIOPort  Port=10  Side=Left
  Moment : PMIOPort  Port=11  Side=Left
  Moment1 : PMIOPort  Port=12  Side=Left
  Moment2 : PMIOPort  Port=13  Side=Left
  Moment3 : PMIOPort  Port=14  Side=Left
  Rotation10 : PMIOPort  Port=15  Side=Left
  Rotation11 : PMIOPort  Port=16  Side=Left
  Rotation12 : PMIOPort  Port=17  Side=Left
  Rotation13 : PMIOPort  Port=18  Side=Left
  Moment4 : PMIOPort  Port=19  Side=Left
  Moment5 : PMIOPort  Port=20  Side=Left
  Moment6 : PMIOPort  Port=21  Side=Left
  Moment7 : PMIOPort  Port=22  Side=Left
  Moment8 : PMIOPort  Port=23  Side=Left
  Rotation14 : PMIOPort  Port=24  Side=Left
  Moment9 : PMIOPort  Port=25  Side=Left
  Moment10 : PMIOPort  Port=26  Side=Left
  Moment11 : PMIOPort  Port=27  Side=Left
  Moment12 : PMIOPort  Port=28  Side=Left
  Moment13 : PMIOPort  Port=29  Side=Left
  Moment14 : PMIOPort  Port=30  Side=Left
  L5-S1 FE Simscape Rotation : Outport
  L4-L5 FE Simscape Rotation : Outport  Port=2
  L3-L4 FE Simscape Rotation : Outport  Port=3
  L2-L3 FE Simscape Rotation : Outport  Port=4
  L5-S1 FE Simscape Moment : Outport  Port=5
  L4-L5 FE Simscape Moment : Outport  Port=6
  L3-L4 FE Simscape Moment : Outport  Port=7
  L2-L3 FE Simscape Moment : Outport  Port=8
  L1-L2 FE Simscape Rotation : Outport  Port=9
  L1-L2 FE Simscape Moment : Outport  Port=10
  L2-L3 LB Simscape Rotation : Outport  Port=11
  L5-S1 LB Simscape Rotation : Outport  Port=12
  L4-L5 LB Simscape Rotation : Outport  Port=13
  L2-L3 LB Simscape Moment : Outport  Port=14
  L1-L2 LB Simscape Rotation : Outport  Port=15
  L3-L4 LB Simscape Rotation : Outport  Port=16
  L5-S1 LB Simscape Moment : Outport  Port=17
  L4-L5 LB Simscape Moment : Outport  Port=18
  L1-L2 LB Simscape Moment : Outport  Port=19
  L3-L4 LB Simscape Moment : Outport  Port=20
  L2-L3 AR Simscape Rotation : Outport  Port=21
  L2-L3 AR Simscape Moment : Outport  Port=22
  L1-L2 AR Simscape Rotation : Outport  Port=23
  L5-S1 AR Simscape Rotation : Outport  Port=24
  L4-L5 AR Simscape Rotation : Outport  Port=25
  L1-L2 AR Simscape Moment : Outport  Port=26
  L3-L4 AR Simscape Rotation : Outport  Port=27
  L5-S1 AR Simscape Moment : Outport  Port=28
  L4-L5 AR Simscape Moment : Outport  Port=29
  L3-L4 AR Simscape Moment : Outport  Port=30
  wires:
  Subsystem9/1(L1-L2 FE Simscape Rotation) -> L1-L2 FE Simscape Rotation/1
  Subsystem5/1(L3-L4 AR Simscape Rotation) -> L3-L4 AR Simscape Rotation/1
  Subsystem5/2(L3-L4 AR Simscape Moment) -> L3-L4 AR Simscape Moment/1
  Subsystem9/2(L1-L2 FE Simscape Moment) -> L1-L2 FE Simscape Moment/1
  Subsystem/1(L4-L5 FE Simscape Rotation) -> L4-L5 FE Simscape Rotation/1
  Subsystem6/1(L2-L3 FE Simscape Rotation) -> L2-L3 FE Simscape Rotation/1
  L5-S1 FE setup/1(L5-S1 FE Simscape Rotation) -> L5-S1 FE Simscape Rotation/1
  Subsystem6/2(L2-L3 FE Simscape Moment) -> L2-L3 FE Simscape Moment/1
  Subsystem3/1(L3-L4 FE Simscape Rotation) -> L3-L4 FE Simscape Rotation/1
  L5-S1 FE setup/2(L5-S1 FE Simscape Moment) -> L5-S1 FE Simscape Moment/1
  Subsystem4/1(L3-L4 LB Simscape Rotation) -> L3-L4 LB Simscape Rotation/1
  Subsystem2/1(L4-L5 AR Simscape Rotation) -> L4-L5 AR Simscape Rotation/1
  L5-S1 AR setup/1(L5-S1 AR Simscape Rotation) -> L5-S1 AR Simscape Rotation/1
  L5-S1 AR setup/2(L5-S1 AR Simscape Moment) -> L5-S1 AR Simscape Moment/1
  Subsystem/2(L4-L5 FE Simscape Moment) -> L4-L5 FE Simscape Moment/1
  Subsystem11/1(L1-L2 AR Simscape Rotation) -> L1-L2 AR Simscape Rotation/1
  L5-S1 LB setup/2(L5-S1 LB Simscape Moment) -> L5-S1 LB Simscape Moment/1
  Subsystem3/2(L3-L4 FE Simscape Moment) -> L3-L4 FE Simscape Moment/1
  Subsystem8/2(L2-L3 AR Simscape Moment) -> L2-L3 AR Simscape Moment/1
  Subsystem8/1(L2-L3 AR Simscape Rotation) -> L2-L3 AR Simscape Rotation/1
  Subsystem7/2(L2-L3 LB Simscape Moment) -> L2-L3 LB Simscape Moment/1
  Subsystem7/1(L2-L3 LB Simscape Rotation) -> L2-L3 LB Simscape Rotation/1
  L5-S1 LB setup/1(L5-S1 LB Simscape Rotation) -> L5-S1 LB Simscape Rotation/1
  Subsystem1/1(L4-L5 LB Simscape Rotation) -> L4-L5 LB Simscape Rotation/1
  Subsystem4/2(L3-L4 LB Simscape Moment) -> L3-L4 LB Simscape Moment/1
  Subsystem1/2(L4-L5 LB Simscape Moment) -> L4-L5 LB Simscape Moment/1
  Subsystem10/2(L1-L2 LB Simscape Moment) -> L1-L2 LB Simscape Moment/1
  Subsystem2/2(L4-L5 AR Simscape Moment) -> L4-L5 AR Simscape Moment/1
  Subsystem11/2(L1-L2 AR Simscape Moment) -> L1-L2 AR Simscape Moment/1
  Subsystem10/1(L1-L2 LB Simscape Rotation) -> L1-L2 LB Simscape Rotation/1
  connections:
  Moment6/RConn1 -- Subsystem2/LConn1
  Rotation/RConn1 -- Subsystem9/LConn2
  Moment3/RConn1 -- Subsystem7/LConn1
  Moment8/RConn1 -- Subsystem8/LConn1
  Rotation4/RConn1 -- Subsystem3/LConn2
  Rotation1/RConn1 -- Subsystem6/LConn2
  Moment7/RConn1 -- Subsystem5/LConn1
  Rotation14/RConn1 -- Subsystem11/LConn2
  Rotation9/RConn1 -- Subsystem10/LConn2
  Moment4/RConn1 -- Subsystem10/LConn1
  Rotation5/RConn1 -- L5-S1 LB setup/LConn2
  Moment/RConn1 -- L5-S1 LB setup/LConn1
  Moment11/RConn1 -- Subsystem9/LConn1
  Rotation2/RConn1 -- L5-S1 FE setup/LConn2
  Rotation8/RConn1 -- Subsystem7/LConn2
  Rotation13/RConn1 -- Subsystem8/LConn2
  Moment12/RConn1 -- Subsystem3/LConn1
  Moment13/RConn1 -- Subsystem/LConn1
  Moment10/RConn1 -- L5-S1 FE setup/LConn1
  Rotation3/RConn1 -- Subsystem/LConn2
  Moment9/RConn1 -- Subsystem11/LConn1
  Rotation6/RConn1 -- Subsystem1/LConn2
  Moment1/RConn1 -- Subsystem1/LConn1
  Rotation7/RConn1 -- Subsystem4/LConn2
  Moment5/RConn1 -- L5-S1 AR setup/LConn1
  Rotation11/RConn1 -- Subsystem2/LConn2
  Rotation12/RConn1 -- Subsystem5/LConn2
  Moment14/RConn1 -- Subsystem6/LConn1
  Rotation10/RConn1 -- L5-S1 AR setup/LConn2
  Moment2/RConn1 -- Subsystem4/LConn1
